simulink model "closedloopcontrol_veryfirst"  (R2016a)
settings: Solver=FixedStepAuto  StartTime=0.0  StopTime=1  FixedStep=1e-6  RelTol=1e-3
libraries: powerlib x5, electricdrivelib x5, factslib x1, re_lib x1
settings Model: Creator=mesutto  LastModifiedBy=mesutto

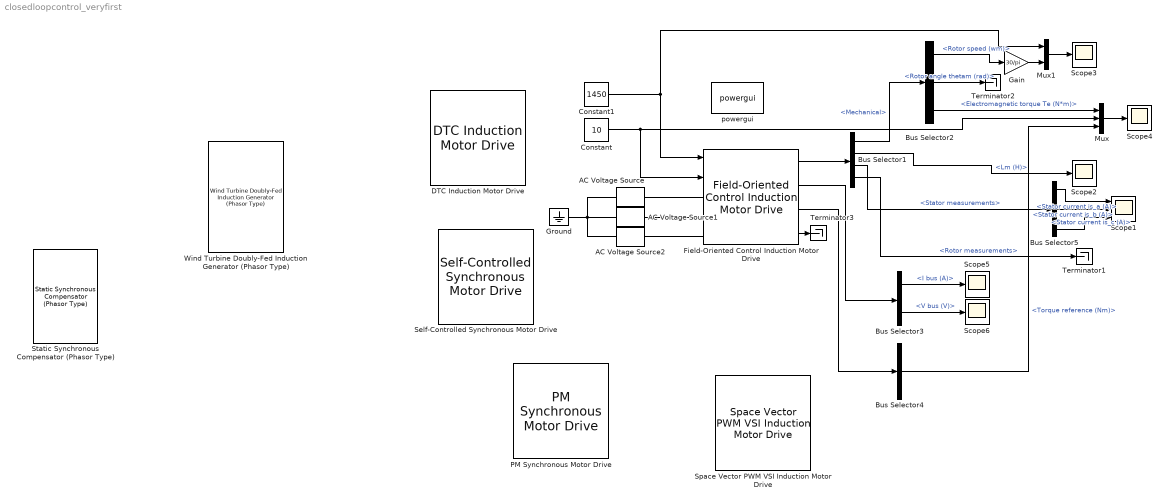
== system closedloopcontrol_veryfirst ==
  AC Voltage Source : powerlib/Electrical Sources/AC Voltage Source  Amplitude=230*sqrt(2)  Phase=0  Frequency=50  SampleTime=0  Measurements=None  BusType=swing  Pref=10e3  Qref=0  Qmin=-inf  Qmax=+inf
  AC Voltage Source1 : powerlib/Electrical Sources/AC Voltage Source  Amplitude=230*sqrt(2)  Phase=-120  Frequency=50  SampleTime=0  Measurements=None  BusType=swing  Pref=10e3  Qref=0  Qmin=-inf  Qmax=+inf
  AC Voltage Source2 : powerlib/Electrical Sources/AC Voltage Source  Amplitude=230*sqrt(2)  Phase=120  Frequency=50  SampleTime=0  Measurements=None  BusType=swing  Pref=10e3  Qref=0  Qmin=-inf  Qmax=+inf
  Bus Selector1 : BusSelector  OutputSignals=Mechanical,Lm (H),Stator measurements,Rotor measurements
  Bus Selector2 : BusSelector  OutputSignals=Rotor speed (wm),Rotor angle thetam (rad),Electromagnetic torque Te (N*m)
  Bus Selector3 : BusSelector  OutputSignals=I bus (A),V bus (V)
  Bus Selector4 : BusSelector  OutputSignals=Torque reference (Nm)
  Bus Selector5 : BusSelector  OutputSignals=Stator current is_a (A),Stator current is_b (A),Stator current is_c (A)
  Constant : Constant  Value=10
  Constant1 : Constant  Value=1450
  DTC Induction Motor Drive : electricdrivelib/AC drives/DTC Induction Motor Drive  showMaskWarnings=on  AverageValue=off  MechanicalLoad=Torque Tm  driveType=AC4  outputBusMode=Multiple output buses  baseSampleTime=0
  Field-Oriented Control Induction Motor Drive : electricdrivelib/AC drives/Field-Oriented Control Induction Motor Drive  showMaskWarnings=on  AverageValue=off  MechanicalLoad=Torque Tm  driveType=AC3  outputBusMode=Multiple output buses  baseSampleTime=1e-06
  Gain : Gain  Gain=30/pi
  Ground : powerlib/Elements/Ground  LConnTagsString=a
  Mux : Mux  Inputs=3
  Mux1 : Mux  Inputs=2
  PM Synchronous Motor Drive : electricdrivelib/AC drives/PM Synchronous Motor Drive  showMaskWarnings=on  AverageValue=off  MechanicalLoad=Torque Tm  driveType=AC6  outputBusMode=Multiple output buses  baseSampleTime=0
  Scope1 : Scope  NumInputPorts=3
  Scope{2..6} (5 alike) : Scope
  Self-Controlled Synchronous Motor Drive : electricdrivelib/AC drives/Self-Controlled Synchronous Motor Drive  showMaskWarnings=off  AverageValue=off  MechanicalLoad=Torque Tm  driveType=AC5  outputBusMode=Multiple output buses  baseSampleTime=0
  Space Vector PWM VSI Induction Motor Drive : electricdrivelib/AC drives/Space Vector PWM VSI Induction Motor Drive  showMaskWarnings=on  AverageValue=off  MechanicalLoad=Torque Tm  driveType=AC2  outputBusMode=Multiple output buses  baseSampleTime=0
  Static Synchronous Compensator (Phasor Type) : factslib/Power-Electronics Based FACTS/Static Synchronous Compensator (Phasor Type)  SystemNominal=[ 500e3, 60 ]  Pnom_SH=100e6  RL_SH=[ 0.22/30, 0.22 ]  Iinit_SH=[0, 0 ]  VnomDC=40000  C_DC=750e-6/2  OpMode_SH=Voltage regulation  Vref_SH=1.00  ExternalVref=off  MaxRateChangeVref_SH=10  Droop_SH=0.03  Par_VacReg=[5, 1000]  Qref_SH=0  MaxRateChangeQref_SH=2  Par_VdcReg=[0.1e-3, 20e-3]  Par_IReg_SH=[0.3, 10, 0.22]
  Terminator1 : Terminator
  Terminator2 : Terminator
  Terminator3 : Terminator
  Wind Turbine Doubly-Fed Induction Generator (Phasor Type) : re_lib/Wind Generation/Wind Turbine Doubly-Fed Induction Generator (Phasor Type)  ExternalTm=off  nom=[1.5e6/0.9 575 60]  sta=[ 0.00706 0.171]  rot=[ 0.005 0.156]  Lm=2.9  mec=[5.04 0.01 3]  init=[0.2 0 0 0 0 0]  speed_power=[0 0; 0.24 0.007; 0.36 0.024; 0.6 0.112; 0.96 0.46; 1.2 0.898; 1.5 0.898]  Pmec=1.5e6  speed_ABCD=[0.7 0.71 1.2 1.21]  power_C=0.73  wind_point_C=12  pitch_gain=500  pitch_max=45  pitch_rate=2  Pmax=0.5  Lchoke=[0.15 0.15/100]  init_inductor=[0 90]  Vdc_nom=1200  capacitor=10000e-6  ControlVQ=Voltage regulation  Vref=1.0  ExternalVref=off  Qref=0  ExternalQref=on  Iq_ref=0  ExternalIqref=off  Kpi_volt_reg=[1.25 300]  Xs=0.02  Kpi_Q=[0.05 5]  Kpi_power_reg=[1 100]  Kpi_dc_reg=[0.002 0.05]  Kpi_grid_side_cur_reg=[1 100]  Kpi_rotor_side_cur_reg=[0.3 8]  V_slew_rate=100  Q_slew_rate=100  power_slew_rate=1  current_slew_rate=200
  powergui : powerlib/powergui  Priority=1  SimulationMode=Discrete  SolverType=Tustin/Backward Euler (TBE)  SampleTime=1e-6  frequency=60  SPID=off  DisableSnubberDevices=off  DisableRonSwitches=off  DisableVfSwitches=off  SwTol=0  DisplayEquations=off  Interpol=off  ExternalGateDelay=off  methode=off  Ts=10  FunctionMessages=off  echomessages=off  HookPort=off  EnableUseOfTLC=off  x0status=blocks  frequencyindice=50  Pbase=100e6  ErrMax=1e-4  Iterations=50  UnitsV=kV  UnitsW=MW  buscounter=0  RestoreLinks=warning  ResistiveCurrentMeasurement=off  Frange=[0:2:500]  Ylog=off  Xlog=on  ShowGrid=off  save=off  variable=ZData  structure=0  ZoomFFT=off  StartTime=0.0  cycles=1  DisplayStyle=1  fundamental=60  FreqAxis=off  MaxFrequency=1000  frequencyindicesteady=1  RmsSteady=1  display=off
  wires:
  Field-Oriented Control Induction Motor Drive/1 -> Bus Selector1/1
  Bus Selector1/1 -> Bus Selector2/1  "<Mechanical>"
  Bus Selector2/2 -> Terminator2/1  "<Rotor angle thetam (rad)>"
  Bus Selector1/2 -> Scope2/1  "<Lm (H)>"
  Bus Selector1/3 -> Bus Selector5/1  "<Stator measurements>"
  Bus Selector1/4 -> Terminator1/1  "<Rotor measurements>"
  Constant/1 -> Mux/2, Field-Oriented Control Induction Motor Drive/2
  Constant1/1 -> Field-Oriented Control Induction Motor Drive/1, Mux1/1
  Mux/1 -> Scope4/1
  Bus Selector2/3 -> Mux/1  "<Electromagnetic torque Te (N*m)>"
  Field-Oriented Control Induction Motor Drive/2 -> Bus Selector3/1
  Bus Selector3/1 -> Scope5/1  "<I bus (A)>"
  Bus Selector3/2 -> Scope6/1  "<V bus (V)>"
  Field-Oriented Control Induction Motor Drive/3 -> Bus Selector4/1
  Field-Oriented Control Induction Motor Drive/4 -> Terminator3/1
  Bus Selector4/1 -> Mux/3  "<Torque reference (Nm)>"
  Mux1/1 -> Scope3/1
  Bus Selector2/1 -> Gain/1  "<Rotor speed (wm)>"
  Gain/1 -> Mux1/2
  Bus Selector5/1 -> Scope1/1  "<Stator current is_a (A)>"
  Bus Selector5/2 -> Scope1/2  "<Stator current is_b (A)>"
  Bus Selector5/3 -> Scope1/3  "<Stator current is_c (A)>"
  connections:
  AC Voltage Source/RConn1 -- Field-Oriented Control Induction Motor Drive/LConn1
  Field-Oriented Control Induction Motor Drive/LConn2 -- AC Voltage Source1/RConn1
  AC Voltage Source2/RConn1 -- Field-Oriented Control Induction Motor Drive/LConn3
  Ground/LConn1 -- AC Voltage Source2/LConn1 -- AC Voltage Source/LConn1 -- AC Voltage Source1/LConn1
